simulink model "LED"  (R2022b)
settings: Solver=FixedStepDiscrete  StartTime=0.0  StopTime=inf  FixedStep=0.1  RelTol=1e-3
PreLoadFcn:
  | canMessageBusType;
  | canFDMessageBusType;
libraries: simulink x8, canfdmsglib x2
PreSaveFcn:
  | filename = 'LED';
  | dictionaryObj  = Simulink.data.dictionary.open([filename,'.sldd']);
  | saveChanges(dictionaryObj);
  | close(dictionaryObj);
  | disp([filename,'.sldd 已保存']);
settings Model: DataDictionary=LED.sldd  Creator=Ligoo  LastModifiedBy=CENSORED
settings DataIOCC: SaveOutput=off  SignalLogging=off  DSMLogging=off  SaveTime=off  ReturnWorkspaceOutputs=off
settings OptimizationCC: DefaultParameterBehavior=Inlined  DefaultUnderspecifiedDataType=single  EnableMemcpy=off  ActiveStateOutputEnumStorageType=uint16  ZeroExternalMemoryAtStartup=off  ZeroInternalMemoryAtStartup=off  NoFixptDivByZeroProtection=on  EfficientFloat2IntCast=on  LifeSpan=Inf  MaxStackSize=200  OptimizeBlockOrder=speed  DifferentSizesBufferReuse=on  EfficientTunableParamExpr=on
settings DebuggingCC: SignalInfNanChecking=error  SignalRangeChecking=warning  AlgebraicLoopMsg=error  MergeDetectMultiDrivingBlocksExec=none  TasksWithSamePriorityMsg=error  IntegerOverflowMsg=error  UnconnectedInputMsg=error  UnconnectedOutputMsg=error  UnconnectedLineMsg=error  UniqueDataStoreMsg=warning  ModelReferenceIOMsg=error  ModelReferenceVersionMismatchMessage=error  StateNameClashWarn=warning  SFUnexpectedBacktrackingDiag=warning  SFNoUnconditionalDefaultTransitionDiag=warning  SFUndirectedBroadcastEventsDiag=error  IntegerSaturationMsg=error
settings HardwareCC: ProdBitPerPointer=32  ProdBitPerSizeT=32  ProdBitPerPtrDiffT=32  ProdLargestAtomicInteger=Long  ProdWordSize=32  ProdHWDeviceType=ARM Compatible->ARM 7
settings ModelReferenceCC: EnableRefExpFcnMdlSchedulingChecks=on
settings SFSimCC: MATLABDynamicMemAlloc=off
settings SFSimCC: SimCustomHeaderCode=|
  | #include "LED_Ctrl.h"
  | #include "ADC_userCode.h"
settings SFSimCC: SimUserSources=|
  | LED_Ctrl.c
  | ADC_userCode.c
settings RTWCC: Description=Embedded Coder  SystemTargetFile=ert.tlc  GenCodeOnly=on  TemplateMakefile=ert_default_tmf  GenerateReport=on  RTWUseSimCustomCode=on  Toolchain=LCC-win64 v2.4.1 | gmake (64-bit Windows)  IncludeHyperlinkInReport=on  LaunchReport=on  GenerateTraceInfo=on  GenerateTraceReport=on  GenerateTraceReportSl=on  GenerateTraceReportSf=on  GenerateTraceReportEml=on
settings RTWCC: CustomHeaderCode=|
  | #include "LED_Ctrl.h"
  | #include "ADC_userCode.h"
settings RTWCC: CustomSource=|
  | LED_Ctrl.c
  | ADC_userCode.c
settings CodeAppCC: ForceParamTrailComments=on  IgnoreCustomStorageClasses=off  OperatorAnnotations=on  SimulinkDataObjDesc=on  SFDataObjDesc=on  MATLABFcnDesc=on  CustomSymbolStrUtil=$R$N$C  InsertBlockDesc=on  MATLABSourceComments=on
settings ERTTargetCC: MultiwordLength=2048  ConcurrentExecutionCompliant=off  IncludeMdlTerminateFcn=off  SuppressErrorStatus=on  SupportAbsoluteTime=off  SupportNonFinite=off  SupportComplex=off  ModelStepFunctionPrototypeControlCompliant=off  CPPClassGenCompliant=off  ArrayLayout=Row-major  GenerateASAP2=on  InlinedParameterPlacement=NonHierarchical  ERTCustomFileTemplate=example_file_process.tlc
settings ConfigComp: CovSaveCumulativeToWorkspaceVar=on  CovSaveSingleToWorkspaceVar=on  CovExternalEMLEnable=off  DVTestSuiteOptimization=CombinedObjectives (Nonlinear Extended)  DVDetectActiveLogic=on  DVModelReferenceHarness=on  DVHarnessSource=Signal Editor

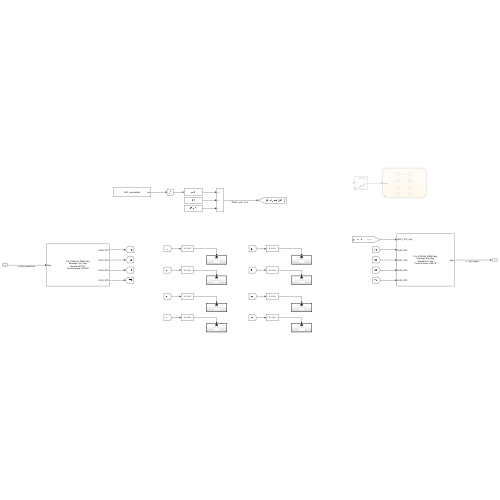
[thumbnail: Simulink's stored preview of the top-level diagram]
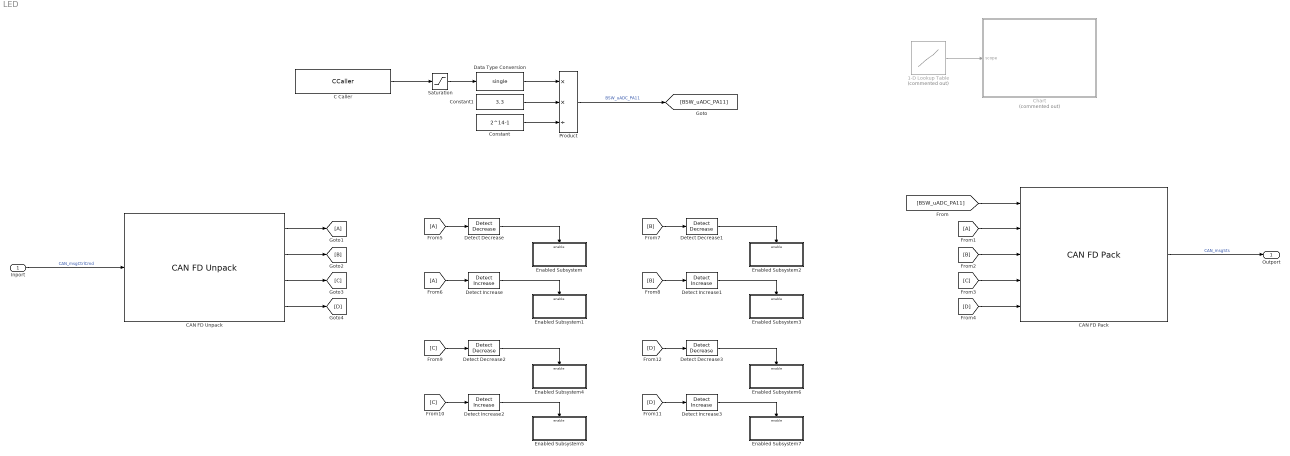
== system LED ==
  Inport : Inport  OutDataTypeStr=Bus: CAN_FD_MESSAGE_BUS  BusOutputAsStruct=on
  1-D Lookup Table : Lookup_n-D  Commented=on  NumberOfTableDimensions=1  BreakpointsForDimension1=[0:1:2:3]  Table=[1:2:3:4]  InterpMethod=Flat  ExtrapMethod=Clip  InternalRulePriority=Speed  OutDataTypeStr=uint8  RndMeth=Simplest
  C Caller : CCaller  FunctionName=ADC_userGetAdc  PortSpecificationStruct="%)30     .    & (   8    (     @         %    \"     $    !     0         %  0 \"0    $    _    07)G3F%M90  4&]R=$YA;64 4V-O<&4     26YD97@     5'EP90      4VEZ90      27-';&]B86P   X    P    !@    @    $          4    (     0    ,    !         !   P!O=70 #@   #     &    \"     0         !0    @    !     P    $         $  # &]U=  .    .     8    (    !          %    \"     $    &     0         0    !@   $]U='!U=   #@   #@    &    \"     8         !0    @    !     0    $         \"0    @               X    X    !@    @    $          4    (     0    8    !         !     &    =6EN=#$V   .    ,     8    (    !          %    \"     $    !     0         0  $ ,0    X    P    !@    @    ) @        4    (     0    $    !          (  0"
  CAN FD Pack : canfdmsglib/CAN FD Pack  CANdbFile=D:\S32K344_DEMO2\S32K344_DEMO.dbc  MsgList=Sts_Meg  MsgName=Sts_Meg  ProtocolMode=CAN FD  MsgIDType=Standard (11-bit identifier)  MsgIdentifier=258  MsgLength=8  Remote=off  BRSSwitch=on  ApplyMinMax=off  SignalInfo={'ADC1_S10_Vltg','16','16','BE','unsigned','Standard','0','0.001','0','-Inf','Inf';'LED0_STS','0','1','BE','unsigned','Standard','0','1','0','-Inf','Inf';'LED1_STS','3','1','BE','unsigned','Standard','0','1','0','-Inf','Inf';'LED2_STS','1','1','BE','unsigned','Standard','0','1','0','-Inf','Inf';'LED3_STS','2','1','BE','unsigned','Standard','0','1','0','-Inf','Inf'}
      settings: DataFormat=CANdb specified signals
  CAN FD Unpack : canfdmsglib/CAN FD Unpack  CANdbFile=D:\S32K344_DEMO2\S32K344_DEMO.dbc  MsgList=Ctrl_Cmd  MsgName=Ctrl_Cmd  ProtocolMode=CAN FD  MsgIDType=Standard (11-bit identifier)  MsgIdentifier=257  MsgLength=8  SignalInfo={'LED0_STS','0','1','BE','unsigned','Standard','0','1','0','-Inf','Inf';'LED1_STS','6','1','BE','unsigned','Standard','0','1','0','-Inf','Inf';'LED2_STS','2','1','BE','unsigned','Standard','0','1','0','-Inf','Inf';'LED3_STS','3','1','BE','unsigned','Standard','0','1','0','-Inf','Inf'}  IDPort=off  TimestampPort=off  ErrorPort=off  RemotePort=off  LengthPort=off  StatusPort=off  BRSPort=off  ESIPort=off  DLCPort=off  ApplyMinMax=off
      settings: DataFormat=CANdb specified signals
  Chart : Stateflow chart  Commented=on  TreatAsAtomicUnit=on
  Constant : Constant  Value=2^14-1  OutDataTypeStr=single
  Constant1 : Constant  Value=3.3  OutDataTypeStr=single
  Data Type Conversion : DataTypeConversion  OutDataTypeStr=single  SaturateOnIntegerOverflow=off  RndMeth=Floor
  Detect Decrease{,1..3} (4 alike) : simulink/Logic and Bit Operations/Detect Decrease  vinit=0.0  OutDataTypeStr=boolean
  Detect Increase{,1..3} (4 alike) : simulink/Logic and Bit Operations/Detect Increase  vinit=0.0  OutDataTypeStr=boolean
  Enabled Subsystem : Subsystem  TreatAsAtomicUnit=on
  Enabled Subsystem1 : Subsystem  TreatAsAtomicUnit=on
  Enabled Subsystem2 : Subsystem  TreatAsAtomicUnit=on
  Enabled Subsystem3 : Subsystem  TreatAsAtomicUnit=on
  Enabled Subsystem4 : Subsystem  TreatAsAtomicUnit=on
  Enabled Subsystem5 : Subsystem  TreatAsAtomicUnit=on
  Enabled Subsystem6 : Subsystem  TreatAsAtomicUnit=on
  Enabled Subsystem7 : Subsystem  TreatAsAtomicUnit=on
  From1 : From
  From5 : From
  From6 : From
  Goto1 : Goto
  Product : Product  Inputs=**/
  Saturation : Saturate  UpperLimit=2^14-1
  Outport : Outport
  wires:
  1-D Lookup Table/1 -> Chart/1(scope)
  Product/1 -> [BSW_uADC_PA11]  "BSW_uADC_PA11"
  C Caller/1 -> Saturation/1
  Data Type Conversion/1 -> Product/1
  Constant/1 -> Product/3
  Constant1/1 -> Product/2
  Saturation/1 -> Data Type Conversion/1
  [BSW_uADC_PA11] -> CAN FD Pack/1
  Inport/1 -> CAN FD Unpack/1  "CAN_msgCtrlCmd"
  CAN FD Unpack/1 -> Goto1/1
  CAN FD Unpack/2 -> [B]
  CAN FD Unpack/3 -> [C]
  CAN FD Unpack/4 -> [D]
  From1/1 -> CAN FD Pack/2
  [B] -> CAN FD Pack/3
  [C] -> CAN FD Pack/4
  [D] -> CAN FD Pack/5
  CAN FD Pack/1 -> Outport/1  "CAN_msgSts"
  From5/1 -> Detect Decrease/1
  Detect Decrease/1 -> Enabled Subsystem/Enable
  From6/1 -> Detect Increase/1
  Detect Increase/1 -> Enabled Subsystem1/Enable
  Detect Increase1/1 -> Enabled Subsystem3/Enable
  [B] -> Detect Increase1/1
  Detect Decrease1/1 -> Enabled Subsystem2/Enable
  [B] -> Detect Decrease1/1
  Detect Increase2/1 -> Enabled Subsystem5/Enable
  [C] -> Detect Increase2/1
  Detect Decrease2/1 -> Enabled Subsystem4/Enable
  [C] -> Detect Decrease2/1
  [D] -> Detect Decrease3/1
  Detect Decrease3/1 -> Enabled Subsystem6/Enable
  [D] -> Detect Increase3/1
  Detect Increase3/1 -> Enabled Subsystem7/Enable

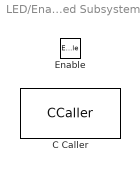
== system LED/Enabled Subsystem ==
  Enable : EnablePort
  C Caller : CCaller  FunctionName=LED0_OFF

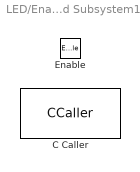
== system LED/Enabled Subsystem1 ==
  Enable : EnablePort
  C Caller : CCaller  FunctionName=LED0_ON

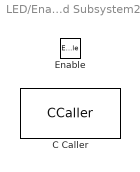
== system LED/Enabled Subsystem2 ==
  Enable : EnablePort
  C Caller : CCaller  FunctionName=LED1_OFF

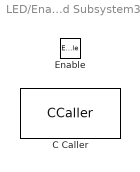
== system LED/Enabled Subsystem3 ==
  Enable : EnablePort
  C Caller : CCaller  FunctionName=LED1_ON

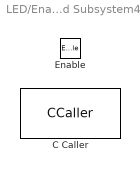
== system LED/Enabled Subsystem4 ==
  Enable : EnablePort
  C Caller : CCaller  FunctionName=LED2_OFF

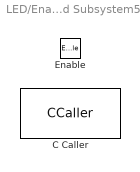
== system LED/Enabled Subsystem5 ==
  Enable : EnablePort
  C Caller : CCaller  FunctionName=LED2_ON

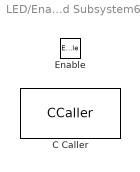
== system LED/Enabled Subsystem6 ==
  Enable : EnablePort
  C Caller : CCaller  FunctionName=LED3_OFF

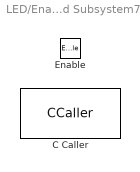
== system LED/Enabled Subsystem7 ==
  Enable : EnablePort
  C Caller : CCaller  FunctionName=LED3_ON

== stateflow chart LED/Chart ==
  state LED0_ON
    en:
    LED0_ON();
  state LED0_OFF
    en:
    LED0_OFF();
  state LED1_ON
    en:
    LED1_ON();
  state LED1_OFF
    en:
    LED1_OFF();
  state LED2_ON
    en:
    LED2_ON();
  state LED2_OFF
    en:
    LED2_OFF();
  state LED3_ON
    en:
    LED3_ON();
  state LED3_OFF
    en:
    LED3_OFF();
  (default) -> LED0_ON
  LED0_OFF -> LED0_ON : [after(1,sec)]
  LED0_ON -> LED0_OFF [order 2] : [scope == 1 &&...
      | after(1,sec)]
  LED0_ON -> LED1_ON [order 1] : [scope > 1&&...
      | after(1,sec)]
  LED1_OFF -> LED0_OFF : [after(1,sec)]
  LED1_ON -> LED1_OFF [order 2] : [scope == 2&&...
      | after(1,sec)]
  LED1_ON -> LED2_ON [order 1] : [scope > 2&&...
      | after(1,sec)]
  LED2_OFF -> LED1_OFF : [after(1,sec)]
  LED2_ON -> LED2_OFF [order 2] : [scope == 3&&...
      | after(1,sec)]
  LED2_ON -> LED3_ON [order 1] : [scope > 3&&...
      | after(1,sec)]
  LED3_OFF -> LED2_OFF : [after(1,sec)]
  LED3_ON -> LED3_OFF : [after(1,sec)]
  data: scope input uint8
